simulink model "SimulacionTanque2"  (R2020a)
settings: Solver=VariableStepAuto  StartTime=0.0  StopTime=tsim  RelTol=1e-3
values from neighbouring files (symbols this model uses):
  alpha = 1    [ParametrosTanque.m]
  Area = 1    [ParametrosTanque.m]
  K1 = 1    [ParametrosTanque.m]
  K2 = K1    (= 1)    [ParametrosTanque.m]
  Kp = .01    (= 0.01)    [ParametrosTanque.m]
  T1 = 90    [ParametrosTanque.m]
  T2 = 10    [ParametrosTanque.m]
  tau1 = 5    [ParametrosTanque.m]
  tau2 = 4    [ParametrosTanque.m]
  tdelay1 = 2 * tmuestra    (= 1)    [ParametrosTanque.m]
  tdelay2 = tmuestra    (= 0.5)    [ParametrosTanque.m]
  tdelayQ = tmuestra    (= 0.5)    [ParametrosTanque.m]
  Te = 45    [ParametrosTanque.m]
  tmuestra = 0.5    [ParametrosTanque.m]
  tvar1 = 23    [ParametrosSimulacion.mat]
  tvar2 = 24    [ParametrosSimulacion.mat]
undefined symbols (not defined in the file or in its folder): seed
settings Model: Creator=pablo  LastModifiedBy=pablo

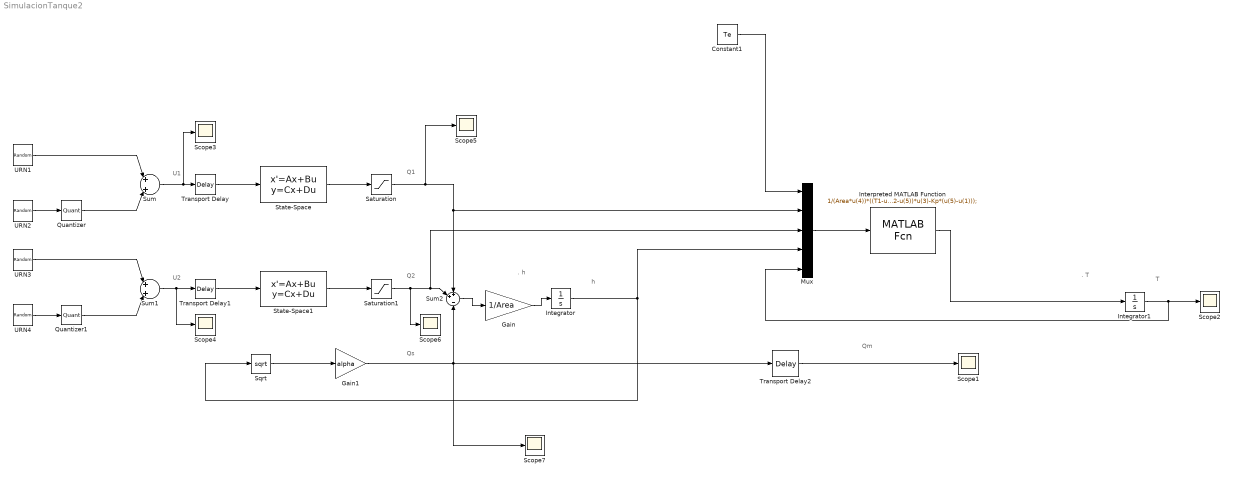
== system SimulacionTanque2 ==
  note: T
  note: Qm
  note: h
  note: U1
  note: .
      |  h
  note: Q1
  note: .
      | T
  note: Q2
  note: U2
  note: Qs
  Constant1 : Constant  Value=Te
  Gain : Gain  Gain=1/Area
  Gain1 : Gain  Gain=alpha
  Integrator : Integrator  InitialCondition=(4/alpha^2)  LimitOutput=on  LowerSaturationLimit=0
  Integrator1 : Integrator  InitialCondition=49.9  LowerSaturationLimit=0
  Interpreted MATLAB Function : MATLABFcn  MATLABFcn=1/(Area*u(4))*((T1-u(5))*u(2)+(T2-u(5))*u(3)-Kp*(u(5)-u(1)));  OutputDimensions=1
  Mux : Mux  Inputs=5
  Quantizer : Quantizer  QuantizationInterval=.25
  Quantizer1 : Quantizer  QuantizationInterval=.25
  Saturation : Saturate  UpperLimit=inf  LowerLimit=0
  Saturation1 : Saturate  UpperLimit=inf  LowerLimit=0
  Scope{1..7} (7 alike) : Scope
  Sqrt : Sqrt  SaturateOnIntegerOverflow=on
  State-Space : StateSpace  A=-1/tau1  B=K1/tau1  D=0  InitialCondition=2
  State-Space1 : StateSpace  A=-1/tau2  B=K2/tau2  D=0  InitialCondition=2
  Sum : Sum  Inputs=|+|+|
  Sum1 : Sum  Inputs=|+|+|
  Sum2 : Sum  Inputs=++|-
  Transport Delay : TransportDelay  DelayTime=tdelay1  InitialOutput=2
  Transport Delay1 : TransportDelay  DelayTime=tdelay2  InitialOutput=2
  Transport Delay2 : TransportDelay  DelayTime=tdelayQ  InitialOutput=4
  URN1 : UniformRandomNumber  Minimum=-.25  Maximum=.25  Seed=seed(1)  SampleTime=tmuestra
  URN2 : UniformRandomNumber  Minimum=.125  Maximum=3.875  Seed=seed(2)  SampleTime=tvar1
  URN3 : UniformRandomNumber  Minimum=-.25  Maximum=.25  Seed=seed(3)  SampleTime=tmuestra
  URN4 : UniformRandomNumber  Minimum=.125  Maximum=3.875  Seed=seed(4)  SampleTime=tvar2
  wires:
  Interpreted MATLAB Function/1 -> Integrator1/1
  Mux/1 -> Interpreted MATLAB Function/1
  Sum2/1 -> Gain/1
  Sqrt/1 -> Gain1/1
  Integrator1/1 -> Mux/5, Scope2/1
  State-Space/1 -> Saturation/1
  Gain1/1 -> Scope7/1, Sum2/3, Transport Delay2/1
  Sum/1 -> Scope3/1, Transport Delay/1
  Transport Delay2/1 -> Scope1/1
  Saturation/1 -> Scope5/1, Mux/2, Sum2/1
  Saturation1/1 -> Scope6/1, Mux/3, Sum2/2
  Gain/1 -> Integrator/1
  Integrator/1 -> Sqrt/1, Mux/4
  Transport Delay/1 -> State-Space/1
  State-Space1/1 -> Saturation1/1
  Transport Delay1/1 -> State-Space1/1
  Constant1/1 -> Mux/1
  URN4/1 -> Quantizer1/1
  URN3/1 -> Sum1/1
  Sum1/1 -> Scope4/1, Transport Delay1/1
  Quantizer1/1 -> Sum1/2
  URN2/1 -> Quantizer/1
  Quantizer/1 -> Sum/2
  URN1/1 -> Sum/1
